simulink model "kalman"  (R2023a)
settings: Solver=VariableStepAuto  StartTime=0  StopTime=T_e  RelTol=1e-3
libraries: BatteryEstimators x1, spspowerguiLib x1
settings Model: Creator=user  LastModifiedBy=Lenovo

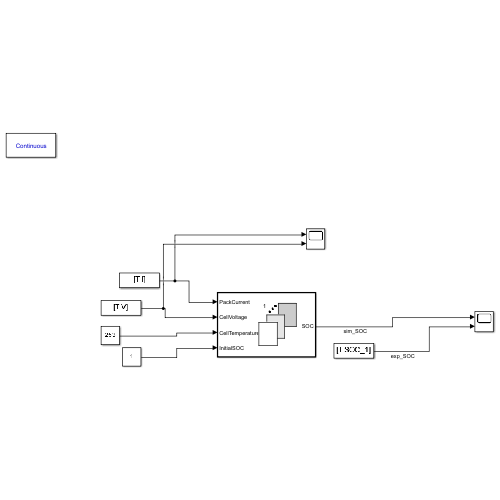
[thumbnail: Simulink's stored preview of the top-level diagram]
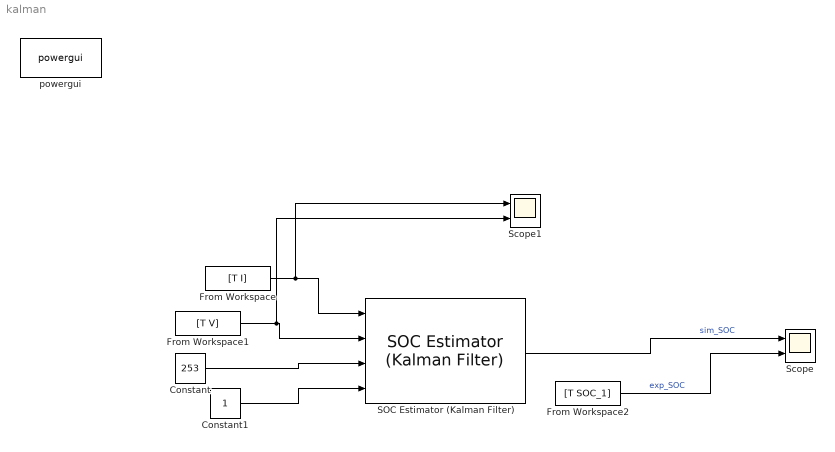
== system kalman ==
  Constant : Constant  Value=253
  Constant1 : Constant
  From Workspace : FromWorkspace  VariableName=[T I]
  From Workspace1 : FromWorkspace  VariableName=[T V]
  From Workspace2 : FromWorkspace  VariableName=[T SOC_1]
  SOC Estimator (Kalman Filter) : BatteryEstimators/SOC Estimator (Kalman Filter)  filterType=Unscented Kalman-Bucy filter  alpha=1  beta=2  kappa=0  Q=|  R=0.1  P0=[1e-5 0; 0 1]  Ts=1  SOC_vec=[.1, .2, .3, .4, .5, .6, .7, .8 , .9, 1]  T_vec=[253, 263, 273, 283, 298]  R0_mat=R0_SOC  R1_mat=R1_SOC  tau1_mat=tau1_SOC  V0_mat=OCV_SOC  AH=2.9
      | [1e-6 0;
      | 0 1e-6]
      settings: LibrarySourceBlock=|
      | batt_sl_lib/Estimators/SOC Estimator
      | (Kalman Filter)
  Scope : Scope  NumInputPorts=2
  Scope1 : Scope  NumInputPorts=2
  powergui : spspowerguiLib/powergui  Priority=1  SimulationMode=Continuous  SampleTime=50e-6  frequency=60  Iterations=50  frequencyindice=60  Pbase=100e6  ErrMax=1e-4  UnitsV=kV  UnitsW=MW  buscounter=0  FunctionMessages=off  echomessages=off  EnableUseOfTLC=off  CurrentSourceSwitches=off  DisableSnubberDevices=off  DisableRonSwitches=off  DisableVfSwitches=off  DisplayEquations=off  AutomaticDiscreteSolvers=off  SolverType=Tustin/Backward Euler (TBE)  Interpol=off  ExternalGateDelay=off  methode=off  Ts=100  x0status=blocks  SPID=on  SwTol=0  HookPort=off  NonlinearTolerance=1e-4  nMaxIteration=100  ContinueOnMaxIteration=off  RestoreLinks=warning  ResistiveCurrentMeasurement=off  Frange=[0:2:500]  Ylog=off  Xlog=on  ShowGrid=off  save=off  variable=ZData  structure=0  ZoomFFT=off  StartTime=0.0  cycles=1  DisplayStyle=1  fundamental=60  FreqAxis=off  MaxFrequency=1000  frequencyindicesteady=1  RmsSteady=1  display=off
  wires:
  From Workspace1/1 -> Scope1/2, SOC Estimator (Kalman Filter)/2
  From Workspace/1 -> Scope1/1, SOC Estimator (Kalman Filter)/1
  Constant/1 -> SOC Estimator (Kalman Filter)/3
  Constant1/1 -> SOC Estimator (Kalman Filter)/4
  SOC Estimator (Kalman Filter)/1 -> Scope/1  "sim_SOC"
  From Workspace2/1 -> Scope/2  "exp_SOC"
